simulink model "cstr_model"  (R2026a)
settings: Solver=ode15s  StopTime=10  MaxStep=0.001  RelTol=1e-6
values from neighbouring files (symbols this model uses):
  CA0 = 0.5    [cstr_worspace.mat]    (also in init_cstr.m)
  CAf = 1.0    (= 1)    [cstr_simulation.m]    (also in cstr_worspace.mat; init_cstr.m)
  Cp = 0.239    [cstr_simulation.m]    (also in cstr_worspace.mat = 1; init_cstr.m)
  deltaH = -5e4    (= -50000)    [cstr_simulation.m]    (also in cstr_worspace.mat = -10; init_cstr.m)
  E_over_R = 8750    [cstr_simulation.m]    (also in cstr_worspace.mat = 1000; init_cstr.m)
  F = 100    [cstr_simulation.m]    (also in cstr_worspace.mat = 1; init_cstr.m)
  k0 = 7.2e10    (= 72000000000)    [cstr_simulation.m]    (also in cstr_worspace.mat = 1; init_cstr.m)
  rho = 1000    [cstr_simulation.m]    (also in cstr_worspace.mat = 1; init_cstr.m)
  T0 = 350    [cstr_worspace.mat]    (also in init_cstr.m)
  Tc = 300    [cstr_simulation.m]    (also in cstr_worspace.mat; init_cstr.m)
  Tf = 350    [cstr_simulation.m]    (also in cstr_worspace.mat; init_cstr.m)
  UA = 5e4    (= 50000)    [cstr_simulation.m]    (also in cstr_worspace.mat = 10; init_cstr.m)
  V = 100    [cstr_simulation.m]    (also in cstr_worspace.mat = 1; init_cstr.m)
settings Model: Creator=Nikhil  LastModifiedBy=Nikhil

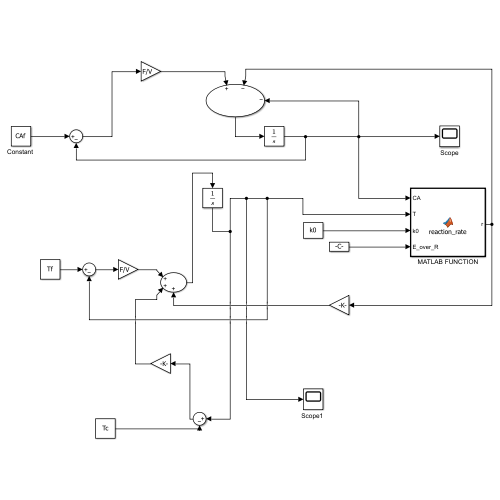
[thumbnail: Simulink's stored preview of the top-level diagram]
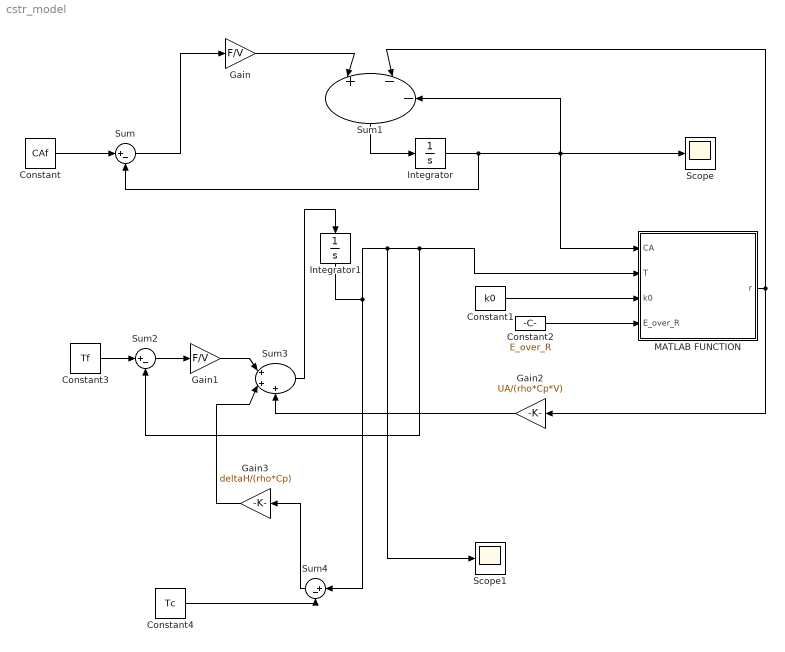
== system cstr_model ==
  "  Scope1   " : Scope
      settings: ActiveDisplayYMinimum=298.88245979868964  ActiveDisplayYMaximum=355.67972668903451
  " Scope " : Scope
      settings: ActiveDisplayYMinimum=0.48964711073549871  ActiveDisplayYMaximum=0.50115032102938906
  "Constant " : Constant  Value=CAf
  Constant1 : Constant  Value=k0
  Constant2 : Constant  Value=E_over_R
  Constant3 : Constant  Value=Tf
  Constant4 : Constant  Value=Tc
  Gain : Gain  Gain=F/V
  Gain1 : Gain  Gain=F/V
  Gain2 : Gain  Gain=UA/(rho*Cp*V)
  Gain3 : Gain  Gain=deltaH/(rho*Cp)
  Integrator : Integrator  InitialCondition=CA0
  Integrator1 : Integrator  InitialCondition=T0
  MATLAB FUNCTION : MATLAB Function  TreatAsAtomicUnit=on
  Sum : Sum  Inputs=|+-
  Sum1 : Sum  Inputs=|+--
  Sum2 : Sum  Inputs=|+-
  Sum3 : Sum  Inputs=|+++
  Sum4 : Sum  Inputs=|+-
  wires:
  "Constant "/1 -> Sum/1
  Constant1/1 -> MATLAB FUNCTION/3(k0)
  Constant2/1 -> MATLAB FUNCTION/4(E_over_R)
  Gain/1 -> Sum1/1
  Sum1/1 -> Integrator/1
  Constant3/1 -> Sum2/1
  Sum2/1 -> Gain1/1
  Gain1/1 -> Sum3/1
  Sum/1 -> Gain/1
  Sum3/1 -> Integrator1/1
  Gain2/1 -> Sum3/3
  Gain3/1 -> Sum3/2
  MATLAB FUNCTION/1(r) -> Sum1/2, Gain2/1
  Integrator1/1 -> "  Scope1   "/1, Sum2/2, MATLAB FUNCTION/2(T), Sum4/1
  Sum4/1 -> Gain3/1
  Constant4/1 -> Sum4/2
  Integrator/1 -> Sum/2, MATLAB FUNCTION/1(CA), " Scope "/1, Sum1/3

== matlab function cstr_model/MATLAB FUNCTION ==
  data: CA input; T input; r output; k0 input; E_over_R input
function r = reaction_rate(CA, T, k0, E_over_R)
% r = k * CA jahan k = k0 * exp(-E_over_R / T)
r = k0 * exp(-E_over_R / T) * CA;
end
